simulink model "full_Model"  (R2022b)
settings: Solver=ode15s  StartTime=0.0  StopTime=400  RelTol=1e-3
InitFcn:
  | ManipulatorSetup
  | init_quad_new_leg_raibert_strategy_v2
values from neighbouring files (symbols this model uses):
  body = 'obstacle'+string(i)    [GUIWithNavigation.m]    (also in RunModel.m)
  endx = 11    [EnvironmentData.mat]    (also in Practice data.mat = 15)
  endy = 11    [EnvironmentData.mat]    (also in Practice data.mat = 14)
  floorl = 20    [EnvironmentData.mat]    (also in GUIWithNavigation.m; Practice data.mat; RunModel.m)
  floorw = 20    [EnvironmentData.mat]    (also in GUIWithNavigation.m; Practice data.mat; RunModel.m)
  planner = plannerRRTStar(ss,stateValidator)    [GUIWithNavigation.m]    (also in RunModel.m)
  startx = 3    [EnvironmentData.mat]    (also in Practice data.mat = 2)
  starty = 3    [EnvironmentData.mat]    (also in Practice data.mat = 2)
  tar1Len = 4    [EnvironmentData.mat]    (also in GUIWithNavigation.m = length(target1); Practice data.mat = 13; RunModel.m = length(target1))
  target = [3 4.43809906251 6.0940682614 6.5 6.5 7.89980588964 9.34167702197 10.6 3 4.34493388975 5.46510729784 7 ... (16 elements, 8x2)]    [EnvironmentData.mat]    (also in GUIWithNavigation.m = cat(1,target1,target2); Practice data.mat = [2 3.44057581018 5.07942513831 5.42542290116 7.21306818311 8; RunModel.m = cat(1,target1,target2))
  tarLen = 8    [EnvironmentData.mat]    (also in RunModel.m = length(target))
undefined symbols (not defined in the file or in its folder): closeFingers, ctrl, Extr_Data_LinkEndHole, grabObjectAngles, grabObjectAngles2, ground, holdFingers, homeAngles, inverseKinematicWeights, l1, l2, m1, m2, openFingers, readyAngles, X, Y, Z
libraries: sm_lib x441, nesl_utility x134, slpidlib x31, robotmaniplib x6, fl_ps_legacy_lib x6, simulink x5, fl_lib x5, Contact_Forces_Lib x4, Parts_Lib x4, sharedtransform x2, dspstat3 x1
(part 15 of 15)

== system full_Model/Manipulator2/Subsystem1/Subsystem7/Subsystem4 ==
  timeValues : Inport
  angleRange : Inport  Port=2
  currentTime : Inport  Port=3
  1-D Lookup Table : Lookup_n-D  NumberOfTableDimensions=1  BreakpointsForDimension1Source=Input port  BreakpointsForDimension1=[-5:5]  TableSource=Input port  Table=tanh([-5:5])  InternalRulePriority=Speed  RndMeth=Simplest
      settings: InputPortMap=u0,p221,p5
  anglePosition : Outport
  wires:
  timeValues/1 -> 1-D Lookup Table/3
  1-D Lookup Table/1 -> anglePosition/1
  currentTime/1 -> 1-D Lookup Table/1
  angleRange/1 -> 1-D Lookup Table/2

== system full_Model/Manipulator2/Subsystem1/Subsystem7/Subsystem5 ==
  timeValues : Inport
  angleRange : Inport  Port=2
  currentTime : Inport  Port=3
  1-D Lookup Table : Lookup_n-D  NumberOfTableDimensions=1  BreakpointsForDimension1Source=Input port  BreakpointsForDimension1=[-5:5]  TableSource=Input port  Table=tanh([-5:5])  InternalRulePriority=Speed  RndMeth=Simplest
      settings: InputPortMap=u0,p221,p5
  anglePosition : Outport
  wires:
  timeValues/1 -> 1-D Lookup Table/3
  1-D Lookup Table/1 -> anglePosition/1
  currentTime/1 -> 1-D Lookup Table/1
  angleRange/1 -> 1-D Lookup Table/2

== system full_Model/Manipulator2/Subsystem1/Subsystem7/Subsystem6 ==
  timeValues : Inport
  angleRange : Inport  Port=2
  currentTime : Inport  Port=3
  1-D Lookup Table : Lookup_n-D  NumberOfTableDimensions=1  BreakpointsForDimension1Source=Input port  BreakpointsForDimension1=[-5:5]  TableSource=Input port  Table=tanh([-5:5])  InternalRulePriority=Speed  RndMeth=Simplest
      settings: InputPortMap=u0,p221,p5
  anglePosition : Outport
  wires:
  timeValues/1 -> 1-D Lookup Table/3
  1-D Lookup Table/1 -> anglePosition/1
  currentTime/1 -> 1-D Lookup Table/1
  angleRange/1 -> 1-D Lookup Table/2

== matlab function full_Model/Controller/QuadCtrl ==
  settings: updateMethod=DISCRETE
  data: fl_ang input; tgt_ctrl_fl output; fr_ang input; rl_ang input; rr_ang input; contact_state input; body_R input; sensing_info input; tgt_ctrl_fr output; tgt_ctrl_rl output; tgt_ctrl_rr output; t input; body parameter; planner parameter; mode input; ctrl_state output; debug output; next_state input
function [tgt_ctrl_fl,tgt_ctrl_fr,tgt_ctrl_rl,tgt_ctrl_rr, ctrl_state, debug] = ...
    controller(fl_ang, fr_ang, rl_ang, rr_ang, ...
    contact_state, body_R, sensing_info, t, body, planner, mode, next_state)

%unpack sensing_info
body_vx = sensing_info(4);
body_vy = sensing_info(5);

% distance from center of mass to shoulder
fl_offset = [body.shoulder_distance;body.y_length/2+body.shoulder_size/2;0];
fr_offset = [body.shoulder_distance;-body.y_length/2-body.shoulder_size/2;0];
rl_offset = [-body.shoulder_distance;body.y_length/2+body.shoulder_size/2;0];
rr_offset = [-body.shoulder_distance;-body.y_length/2-body.shoulder_size/2;0];

%decide state and state transition helpers
persistent state;
persistent timer;
persistent timer2;
if isempty(state)
    state = 0;
end
if isempty(timer)
    timer = 0;
end
if isempty(timer2)
    timer2 = 0;
end

% init variables
           % fl fr rl rr
has_u_ctrl = [1 1 1 1];
normal_virtual_leg1 = [0;0;planner.stand_height];
normal_virtual_leg2 = [0;0;planner.stand_height];
move_fl_end_effector = normal_virtual_leg1;
move_rr_end_effector = normal_virtual_leg1;
move_fr_end_effector = normal_virtual_leg2;
move_rl_end_effector = normal_virtual_leg2;

% turning on spot mechanic
isTurning = mode == 2 || mode == 3;
%{
if isTurning
    leg_a_coef = 1; % -1/3
    leg_b_coef = 1;
else
    leg_a_coef = 1;
    leg_b_coef = 1;
end
%}
leg_a_coef = 1;
leg_b_coef = 1;

% state machine

if state == 0 % standby state
    % in this state, just do nothing, but use time to make sure that all
    % feet stands on the ground

    if contact_state(1) == 1 && contact_state(2) == 1 && contact_state(3) == 1 && contact_state(4) == 1
        %all foot on ground
        if abs(body_vx) < planner.state0_vel_thres 
            timer = timer + 1;
        else
            timer = 0;
        end
        if timer > planner.state0_trans_thres 
            state = 1;
            timer = 0;
        end
    end
elseif state == 1 % swing whole body to get a inital velocity
    timer2 = timer2 + 1;
    move_theta = planner.state0_swing_ang*sin(2*pi/planner.state0_swing_T*timer2);
    move_leg_Rx = [cos(move_theta) 0 sin(move_theta);
        0 1 0;
        -sin(move_theta) 0 cos(move_theta)];
    tgt_virtual_leg1_b = move_leg_Rx*normal_virtual_leg1;
    tgt_virtual_leg2_b = move_leg_Rx*normal_virtual_leg2;
    move_fl_end_effector = tgt_virtual_leg1_b;
    move_rr_end_effector = tgt_virtual_leg1_b;
    move_fr_end_effector = tgt_virtual_leg2_b;
    move_rl_end_effector = tgt_virtual_leg2_b;
        
    if body_vx > planner.state12_trans_speed
        timer = timer + 1;
    else
        timer = 0;
    end
    if timer > 40  %(keep a velocity larger than 0.2 for 0.1s)
        state = next_state;
        timer = 0;
        timer2 = 0;
    end

elseif state == 2 % stance virtual leg1, swing virtual leg2
    timer2 = timer2 + 1;
    if timer2 > planner.leg_swing_time %(0.5s finish movement)
        timer2 = planner.leg_swing_time;
    end
    % stance leg no u control but need to balance the body
               % fl fr rl rr
    has_u_ctrl = [0 1 1 0];
    t = timer2/planner.leg_swing_time;
%     stance_length_coeff = 0.95+0.05*(timer2/planner.leg_swing_time);
    stance_length_coeff = 0.2*t^2 - 0.2*t + 1;
    tgt_virtual_leg1_b = stance_length_coeff*normal_virtual_leg1;
    move_fl_end_effector = tgt_virtual_leg1_b;
    move_rr_end_effector = tgt_virtual_leg1_b;
    
    
    % swing leg must consider body angle 
%     move_theta = -11/180*pi*(t);
    length_coeff = 0.8*t^2-0.8*t+1;
    % move leg in x direction
    move_theta = get_move_angle(length_coeff*normal_virtual_leg2,body_vx, planner.tgt_body_vx, planner);
    
    move_leg_Rx = [cos(move_theta) 0 sin(move_theta);
        0 1 0;
        -sin(move_theta) 0 cos(move_theta)];
    move_leg_Rx2 = [cos(move_theta) 0 sin(move_theta);
        0 1 0;
        -sin(move_theta) 0 cos(move_theta)];
    tgt_virtual_leg2_a = length_coeff*move_leg_Rx2*normal_virtual_leg2;
    tgt_virtual_leg2_b = length_coeff*move_leg_Rx*normal_virtual_leg2;
    
    % move leg in y direction
    sagittal_angle = get_sagittal_angle(tgt_virtual_leg2_b,body_R, body_vy, planner);
    move_leg_Ry =[1 0 0;
                 0 cos(sagittal_angle) -sin(sagittal_angle);
                 0 sin(sagittal_angle) cos(sagittal_angle)];
    tgt_virtual_leg2_b = move_leg_Ry*tgt_virtual_leg2_b;
    tgt_virtual_leg2_a = move_leg_Ry*tgt_virtual_leg2_a;
    
    
    move_fr_end_effector = body_R'*(tgt_virtual_leg2_b+fr_offset)-fr_offset;
    if norm(move_fr_end_effector) > body.max_stretch
        move_fr_end_effector = move_fr_end_effector/norm(move_fr_end_effector)*body.max_stretch;
    end
    move_rl_end_effector = body_R'*(tgt_virtual_leg2_a+rl_offset)-rl_offset;
    if norm(move_rl_end_effector) > body.max_stretch
        move_rl_end_effector = move_rl_end_effector/norm(move_rl_end_effector)*body.max_stretch;
    end
    
    % state transition
%     if timer2 == planner.leg_swing_time
    if timer2 > 0.5*planner.leg_swing_time && contact_state(2) == 1 && contact_state(3) == 1
        timer = timer + 1;
    else
        timer = 0;
    end
    if timer > 5   % to be determined
        state = next_state;
        timer = 0;
        timer2 = 0;
    end
    
elseif state == 3 % swing virtual leg1, stance virtual leg2
    timer2 = timer2 + 1;
    if timer2 > planner.leg_swing_time %(0.5s finish movement)
        timer2 = planner.leg_swing_time;
    end
    % stance leg no u control but need to balance the body
               % fl fr rl rr
    has_u_ctrl = [1 0 0 1];
%     stance_length_coeff = 0.95+0.05*(timer2/planner.leg_swing_time);
    t = timer2/planner.leg_swing_time;
    stance_length_coeff = 0.2*t^2 - 0.2*t + 1;
    tgt_virtual_leg2_b = stance_length_coeff*normal_virtual_leg2;
    move_fr_end_effector = tgt_virtual_leg2_b;
    move_rl_end_effector = tgt_virtual_leg2_b;
    
    % swing leg must consider body angle 
    % theta is a function of forward velocity 
%     move_theta = -11/180*pi*(t);
    length_coeff = 0.8*t^2-0.8*t+1;
    move_theta = get_move_angle(length_coeff*normal_virtual_leg1,body_vx, planner.tgt_body_vx, planner);
    move_leg_Rx = [cos(move_theta*(1-2*isTurning)) 0 sin(move_theta*(1-2*isTurning));
        0 1 0;
        -sin(move_theta*(1-2*isTurning)) 0 cos(move_theta*(1-2*isTurning))];
    move_leg_Rx2 = [cos(move_theta*(1-2*isTurning)) 0 sin(move_theta*(1-2*isTurning));
        0 1 0;
        -sin(move_theta*(1-2*isTurning)) 0 cos(move_theta*(1-2*isTurning))];
    tgt_virtual_leg1_a = length_coeff*move_leg_Rx2*normal_virtual_leg1;
    tgt_virtual_leg1_b = length_coeff*move_leg_Rx*normal_virtual_leg1;
    
    % move leg in y direction
    sagittal_angle = get_sagittal_angle(tgt_virtual_leg1_b,body_R, body_vy, planner);
    move_leg_Ry =[1 0 0;
                 0 cos(sagittal_angle) -sin(sagittal_angle);
                 0 sin(sagittal_angle) cos(sagittal_angle)];
    tgt_virtual_leg1_b = move_leg_Ry*tgt_virtual_leg1_b;
    tgt_virtual_leg1_a = move_leg_Ry*tgt_virtual_leg1_a;
    
    move_fl_end_effector = body_R'*(tgt_virtual_leg1_b+fl_offset)-fl_offset;
    if norm(move_fl_end_effector) > body.max_stretch
        move_fl_end_effector = move_fl_end_effector/norm(move_fl_end_effector)*body.max_stretch;
    end
    move_rr_end_effector = body_R'*(tgt_virtual_leg1_a+rr_offset)-rr_offset;
    if norm(move_rr_end_effector) > body.max_stretch
        move_rr_end_effector = move_rr_end_effector/norm(move_rr_end_effector)*body.max_stretch;
    end
    
    % state transition
%     if timer2 == planner.leg_swing_time
    if timer2 > 0.5*planner.leg_swing_time && contact_state(1) == 1 && contact_state(4) == 1
        timer = timer + 1;
    else
        timer = 0;
    end
    if timer > 5   % to be determined
        state = next_state;
        timer = 0;
        timer2 = 0;
    end
elseif state == 4 % stabalisation
    timer2 = timer2 + 1;
    move_theta = planner.state0_swing_ang*sin(2*pi/planner.state0_swing_T*timer2);
    move_leg_Rx = [cos(move_theta) 0 sin(move_theta);
        0 1 0;
        -sin(move_theta) 0 cos(move_theta)];
    tgt_virtual_leg1_b = move_leg_Rx*normal_virtual_leg1;
    tgt_virtual_leg2_b = move_leg_Rx*normal_virtual_leg2;
    move_fl_end_effector = tgt_virtual_leg1_b;
    move_rr_end_effector = tgt_virtual_leg1_b;
    move_fr_end_effector = tgt_virtual_leg2_b;
    move_rl_end_effector = tgt_virtual_leg2_b;
        
    timer = timer + 1;
    if timer > 40  %(keep a velocity larger than 0.2 for 0.1s)
        state = next_state;
        timer = 0;
        timer2 = 0;
    end
end

%% fl to joint
[inv_s,inv_u,inv_k] = inverse_kinematics(move_fl_end_effector, body);
fl_tgt_ang_s = inv_s; 
fl_tgt_ang_u = inv_u;       
fl_tgt_ang_k = inv_k; 
tgt_ctrl_fl = [fl_tgt_ang_s;fl_tgt_ang_u;fl_tgt_ang_k;has_u_ctrl(1)];

%% fr to joint
[inv_s,inv_u,inv_k] = inverse_kinematics(move_fr_end_effector, body);
fr_tgt_ang_s = inv_s;
fr_tgt_ang_u = inv_u;
fr_tgt_ang_k = inv_k;
tgt_ctrl_fr = [fr_tgt_ang_s;fr_tgt_ang_u;fr_tgt_ang_k;has_u_ctrl(2)];

%% rl to joint
[inv_s,inv_u,inv_k] = inverse_kinematics(move_rl_end_effector, body);
rl_tgt_ang_s = inv_s;
rl_tgt_ang_u = inv_u;
rl_tgt_ang_k = inv_k;
tgt_ctrl_rl = [rl_tgt_ang_s;rl_tgt_ang_u;rl_tgt_ang_k;has_u_ctrl(3)];

%% rr to joint
[inv_s,inv_u,inv_k] = inverse_kinematics(move_rr_end_effector, body);
rr_tgt_ang_s = inv_s;
rr_tgt_ang_u = inv_u;
rr_tgt_ang_k = inv_k; 
tgt_ctrl_rr = [rr_tgt_ang_s;rr_tgt_ang_u;rr_tgt_ang_k;has_u_ctrl(4)];

ctrl_state = state;
debug = timer;

end

function move_angle = get_move_angle(virtual_leg,body_vx, tgt_body_vx, planner)

    distance = body_vx* planner.Ts/2 + planner.Kv*(tgt_body_vx-body_vx);
    
    if distance > 0.5*norm(virtual_leg)
        distance = 0.5*norm(virtual_leg);
    elseif distance < -0.5*norm(virtual_leg)
        distance = -0.5*norm(virtual_leg);
    end
    
    move_angle = asin(distance/norm(virtual_leg));
    if move_angle > 20/180*pi
        move_angle = 20/180*pi;
    elseif move_angle < -20/180*pi
        move_angle = -20/180*pi;
    end
    
end

function move_angle = get_sagittal_angle(virtual_leg,body_R, body_vy, planner)

    distance = body_vy* planner.y_Ts/2 + planner.y_Kv*(0-body_vy);  

    if distance > 0.5*norm(virtual_leg)
        distance = 0.5*norm(virtual_leg);
    elseif distance < -0.5*norm(virtual_leg)
        distance = -0.5*norm(virtual_leg);
    end
    
    move_angle = asin(distance/norm(virtual_leg));
    if move_angle > 20/180*pi
        move_angle = 20/180*pi;
    elseif move_angle < -20/180*pi
        move_angle = -20/180*pi;
    end
    
end

== stateflow chart full_Model/Controller/High Level Mode Stateflow ==
  state ResetPos
    mode=0;
    ManipTask=1;
  state Stationary
    mode=0;
    ManipTask=0;
  state Turning_Right
    mode=2;
  state Walking
    mode=1;
  state Turning_Left
    mode=3;
  Turning_Right -> ResetPos [order 2] : [resetPos==1]{pos_index=pos_index+2}
  Stationary -> ResetPos [order 2] : [resetPos==1]{pos_index=pos_index+2}
  ResetPos -> Stationary : [manipState==5]
  Walking -> ResetPos [order 4] : [resetPos==1]{pos_index=pos_index+2}
  Turning_Left -> ResetPos [order 2] : [resetPos==1]{pos_index=pos_index+2}
  (default) -> Stationary : {pos_index =2 }
  Turning_Left -> Stationary [order 1] : [delta_theta < ang_threshold]
  Turning_Right -> Stationary [order 1] : [delta_theta > -ang_threshold]
  Stationary -> Walking [order 1] : [~target_reached]
  Walking -> Stationary [order 3] : [target_reached]
      | {pos_index = pos_index + 1}
  Walking -> Turning_Right [order 2] : [delta_theta < -ang_threshold]
  Walking -> Turning_Left [order 1] : [delta_theta > ang_threshold]
  data: pos_index output =0; mode output =0; target_reached input; delta_theta input; ang_threshold local =0.2; resetPos input; ManipTask output; manipState input

== stateflow chart full_Model/Controller/Chart ==
  state PathFollowing
    resetPos=0;
  state ManipulatorTask
    resetPos=1;
  (default) -> PathFollowing
  PathFollowing -> ManipulatorTask : [pos_index==tar1Len]
  ManipulatorTask -> PathFollowing : [manipState==5]
  data: pos_index input; tar1Len input; resetPos output; manipState input

== matlab function full_Model/Manipulator2/Ball Tracking and Handling/MATLAB Function1 ==
  data: objectTransform output; x input; y input; z input; aboveObjectTransform output
function [objectTransform,aboveObjectTransform] = fcn(x,y,z)
rotTransform=[1 0 0;0 -1 0;0 0 -1];
F=rotTransform;
xline=F(1,:);
yline=F(2,:);
zline=F(3,:);
objectTransform = [ xline x;yline y;zline z+0.02;0 0 0 1];
aboveObjectTransform = [xline x;yline y;zline z+0.1;0 0 0 1];

== matlab function full_Model/Manipulator1/MATLAB Function ==
  settings: updateMethod=DISCRETE
  data: quadrupedInPosition input; errorVals input; contactForces input; state input; y output; readyAngles input; grabObjectAngles2 input; grabObjectAngles input; openFingers input; closeFingers input; holdFingers input; stateOut output; objectPosition input; aboveObjectPosition input
function [y,stateOut] = fcn(quadrupedInPosition,errorVals,contactForces,state,readyAngles,grabObjectAngles2,grabObjectAngles,openFingers,closeFingers,holdFingers,objectPosition,aboveObjectPosition)

if quadrupedInPosition == 1
    state = int16(state);

    switch state
        case 0
            y = [readyAngles;openFingers];
        case 1

            y = [aboveObjectPosition;openFingers];
        case 2
            y = [objectPosition;openFingers];
        case 3
            y = [objectPosition;closeFingers];
        case 4
            y = [aboveObjectPosition;closeFingers];
        case 5
            y = [readyAngles;closeFingers];
        otherwise
            y = zeros(13,1);
    end
    
    if state == 0 && min(errorVals) >= -0.01 && max(errorVals) <=0.01
        
        stateOut = 1;
        tic;
    elseif state == 1 && min(errorVals) >= -0.01 && max(errorVals) <=0.01 && toc >= 4
        stateOut = 2;
        tic;
    elseif state == 2 && min(errorVals) >= -0.01 && max(errorVals) <=0.01 && toc >= 0.5
        stateOut = 3;
        tic;
    elseif state == 3 && min(contactForces) >= 0.5 && toc >= 1
        toc;
        stateOut = 4;
        tic;
    elseif state == 4 && min(errorVals) >= -0.01 && max(errorVals) <=0.01 && toc >= 10
        stateOut = 5;
    elseif state == 5 && min(errorVals) >= -0.01 && max(errorVals) <=0.01
        stateOut = 5;
    else
        stateOut = double(state);
    end
else
    y = [readyAngles;openFingers];
    stateOut = 0;
end

== matlab function full_Model/Manipulator1/MATLAB Function1 ==
  data: R input; objectTransform output; x input; y input; z input; aboveObjectTransform output
function [objectTransform,aboveObjectTransform] = fcn(R,x,y,z)

objectTransform = [1 0 0 x;0 -1 0 y;0 0 -1 z+0.02;0 0 0 1];
aboveObjectTransform = [1 0 0 x;0 -1 0 y;0 0 -1 z+0.1;0 0 0 1];

== matlab function full_Model/Manipulator2/End Tracking and handling/MATLAB Function1 ==
  data: objectTransform output; x input; y input; z input; aboveObjectTransform output
function [objectTransform,aboveObjectTransform] = fcn(x,y,z)
rotTransform=[1 0 0;0 -1 0;0 0 -1];
F=rotTransform;
xline=F(1,:);
yline=F(2,:);
zline=F(3,:);
objectTransform = [ xline x;yline y;zline z+0.02;0 0 0 1];
aboveObjectTransform = [xline x;yline y;zline z+0.1;0 0 0 1];

== matlab function full_Model/Manipulator2/MATLAB Function ==
  settings: updateMethod=DISCRETE
  data: quadrupedInPosition input; errorVals input; state input; readyAngles input; openFingers input; closeFingers input; objectPosition input; aboveObjectPosition input; endPos input; aboveEndPos input; time input; y output; stateOut output; getBallPos output; getEndPos output; ballGot output
function [y,stateOut,getBallPos,getEndPos,ballGot] = fcn(quadrupedInPosition,errorVals,state,readyAngles,openFingers,closeFingers,objectPosition,aboveObjectPosition,endPos,aboveEndPos,time)

persistent startTime
if isempty(startTime)
    startTime=0;
end

threshold=0.05;
if quadrupedInPosition == 1
    state = int16(state);

    switch state
        case 0
            y = [readyAngles;openFingers];
            getBallPos=0;
            getEndPos=0;
            ballGot=0;
        case 1
            getBallPos=0;
            getEndPos=0;
            y = [aboveObjectPosition;openFingers];
            ballGot=0;
        case 2
            getBallPos=0;
            getEndPos=0;
            y = [objectPosition;openFingers];
            ballGot=0;
        case 3
            getBallPos=0;
            getEndPos=0;
            y = [objectPosition;closeFingers];
            ballGot=0;
        case 4
            getBallPos=0;
            getEndPos=0;
            y = [aboveObjectPosition;closeFingers];
            ballGot=1;
        case 5
            getBallPos=0;
            getEndPos=0;
            y = [readyAngles;closeFingers];
            ballGot=1;
        otherwise
            y = zeros(13,1);
            getBallPos=0;
            getEndPos=0;
            ballGot=0;
    end
    
    if state == 0 && min(errorVals) >= -threshold && max(errorVals) <=threshold
        getBallPos=1;
        stateOut = 1;
        startTime=time;
    elseif state == 1 && min(errorVals) >= -threshold && max(errorVals) <=threshold && (time-startTime) >= 4
        getBallPos=1;
        stateOut = 2;
        startTime=time;
    elseif state == 2  && (time-startTime) >= 4
        stateOut = 3;
        startTime=time;
    elseif state==3 && min(errorVals) >= -threshold && max(errorVals) <=threshold && (time-startTime) >= 4
        stateOut = 4;
        startTime=time;
    elseif state == 4 && min(errorVals) >= -threshold && max(errorVals) <=threshold && (time-startTime) >= 4
        stateOut = 5;
        startTime=time;
    elseif state == 5 && min(errorVals) >= -threshold && max(errorVals) <=threshold && (time-startTime)>=4
        stateOut = 5;
    else
        stateOut = double(state);
    end

elseif quadrupedInPosition == 2

    switch state
        case 5
            y = [readyAngles;closeFingers];
            getBallPos=0;
            getEndPos=0;
            ballGot=1;
        case 6
            getBallPos=0;
            getEndPos=0;
            y = [aboveEndPos;closeFingers];
            ballGot=1;
        case 7
            getBallPos=0;
            getEndPos=0;
            y = [endPos;closeFingers];
            ballGot=1;
        case 8
            getBallPos=0;
            getEndPos=0;
            y = [endPos;openFingers];
            ballGot=1;
        case 9
            getBallPos=0;
            getEndPos=0;
            y = [aboveEndPos;openFingers];
            ballGot=0;
        case 10
            getBallPos=0;
            getEndPos=0;
            y = [readyAngles;openFingers];
            ballGot=0;
        case 11
            getBallPos=0;
            getEndPos=0;
            y = [readyAngles;openFingers];
            ballGot=0;
        otherwise
            y = zeros(13,1);
            getBallPos=0;
            getEndPos=0;
            ballGot=0;
    end
    if state == 5 && min(errorVals) >= -threshold && max(errorVals) <=threshold
        stateOut = 6;
        startTime=time;
    elseif state == 6 && min(errorVals) >= -threshold && max(errorVals) <=threshold && (time-startTime) >= 4
        getEndPos=1;
        stateOut = 7;
        startTime=time;
    elseif state == 7  && (time-startTime) >= 4
        stateOut = 8;
        startTime=time;
    elseif state==8 && min(errorVals) >= -threshold && max(errorVals) <=threshold && (time-startTime) >= 5
        stateOut = 9;
        startTime=time;
    elseif state == 9 && min(errorVals) >= -threshold && max(errorVals) <=threshold && (time-startTime) >= 10
        stateOut = 10;
        startTime=time;
    elseif state == 10 && min(errorVals) >= -threshold && max(errorVals) <=threshold && (time-startTime)>=4
        stateOut = 11;
        startTime=time;
    elseif state == 11 && min(errorVals) >= -threshold && max(errorVals) <=threshold && (time-startTime)>=4
        stateOut = 11;
    else
        stateOut = double(state);
    end
else
    y = [readyAngles;openFingers];
    stateOut = 0;
    getBallPos=0;
    getEndPos=0;
    ballGot=0;
end

== matlab function full_Model/Manipulator2/Subsystem1/Manipulator interpolator ==
  settings: updateMethod=DISCRETE
  data: desiredAngles input size=[7  1]; angleRangeOut output size=[1 14]; currentAngles input size=[7 1]; timeRangeOut output size=[1 14]; time input; debug output
function [angleRangeOut,timeRangeOut,debug]  = manipInterp(desiredAngles,currentAngles,time)

persistent beginState
persistent ready1
persistent ready2
persistent ready3
persistent ready4
persistent ready5
persistent ready6
persistent ready7

% persistent interval
persistent startTime
persistent angleRange
persistent timeRange

if isempty(beginState)
    beginState=transpose(currentAngles);
end

% if isempty(interval)
%     interval=0.01;
% end
if isempty(startTime)
    startTime=10;
end
if isempty(angleRange)
    angleRange=[transpose(currentAngles),transpose(currentAngles)];
end
if isempty(timeRange)
    timeRange=[ones(1,7)*0,ones(1,7)*600];
end
if isempty(ready1)
    ready1=0;
end
if isempty(ready2)
    ready2=0;
end
if isempty(ready3)
    ready3=0;
end
if isempty(ready4)
    ready4=0;
end
if isempty(ready5)
    ready5=0;
end
if isempty(ready6)
    ready6=0;
end
if isempty(ready7)
    ready7=0;
end

%timeSteps=0.01;
transferTime=3;
%calcTime=timeSteps/transferTime;
angleDif=transpose(abs(desiredAngles-currentAngles));
threshold=0.01;
TcurrentAngles=transpose(currentAngles);
if angleDif(1)>=threshold||angleDif(2)>=threshold||angleDif(3)>=threshold||angleDif(4)>=threshold||angleDif(5)>=threshold||angleDif(6)>=threshold||angleDif(7)>=threshold
    if ready1==0&&ready2==0&&ready3==0&&ready4==0&&ready5==0&&ready6==0&&ready7==0
        beginState=transpose(currentAngles);
        %interval=((desiredAngles-beginState)./calcTime);
        startTime=time;
        ready1=1;
        ready2=1;
        ready3=1;
        ready4=1;
        ready5=1;
        ready6=1;
        ready7=1;
        endTime=transferTime+startTime;
        timeRange=[ones(1,7)*startTime,ones(1,7)*endTime];
        angleRange=[beginState,transpose(desiredAngles)];
    end       
end

if angleDif(1)<=threshold
    ready1=0;
    timeRange(1)=0;
    timeRange(8)=600;
    angleRange(1)=TcurrentAngles(1);
    angleRange(8)=TcurrentAngles(1);
end
if angleDif(2)<=threshold
    ready2=0;
    timeRange(2)=0;
    timeRange(9)=600;
    angleRange(2)=TcurrentAngles(2);
    angleRange(9)=TcurrentAngles(2);
end
if angleDif(3)<=threshold
    ready3=0;
    timeRange(3)=0;
    timeRange(10)=600;
    angleRange(3)=TcurrentAngles(3);
    angleRange(10)=TcurrentAngles(3);
end
if angleDif(4)<=threshold
    ready4=0;
    timeRange(4)=0;
    timeRange(11)=600;
    angleRange(4)=TcurrentAngles(4);
    angleRange(11)=TcurrentAngles(4);
end
if angleDif(5)<=threshold
    ready5=0;
    timeRange(5)=0;
    timeRange(12)=600;
    angleRange(5)=TcurrentAngles(5);
    angleRange(12)=TcurrentAngles(5);
end
if angleDif(6)<=threshold
    ready6=0;
    timeRange(6)=0;
    timeRange(13)=600;
    angleRange(6)=TcurrentAngles(6);
    angleRange(13)=TcurrentAngles(6);
end
if angleDif(7)<=threshold
    ready7=0;
    timeRange(7)=0;
    timeRange(14)=600;
    angleRange(7)=TcurrentAngles(7);
    angleRange(14)=TcurrentAngles(7);
end

angleRangeOut=angleRange;
timeRangeOut=timeRange;
debug=angleDif;

== matlab function full_Model/Controller/MATLAB Function1 ==
  settings: updateMethod=DISCRETE
  data: go input; mode output; targets input; tar1Len input; tarLen input; x input; y input; angle input; done output
function [mode,done] = broadside(go,targets,tar1Len,tarLen,x,y,angle)

persistent targetAssigned
if isempty(targetAssigned)
    targetAssigned=0;
end

persistent broadTarget
if isempty(broadTarget)
    broadTarget=[0,0];
end

persistent points
if isempty(points)
    points=0;
end

persistent point1
if isempty(point1)
    point1=[0,0];
end

persistent point2
if isempty(point2)
    point2=[0,0];
end

persistent currentTarget
if isempty(currentTarget)
    currentTarget=[0,0];
end


if go==1||go==2
    if targetAssigned==0
        if go==1
            broadTarget=targets(tar1Len,:);
        elseif go==2
            broadTarget=targets(tarLen,:);
        end
        if y>broadTarget(2)
            spacing=1;
        else
            spacing=-1;
        end
        if x>broadTarget(1)
            points=2;
            point1=[x,broadTarget(2)+spacing];
            point2=[broadTarget(1),broadTarget(2)+spacing];
        else
            points=1;
            point1=[broadTarget(1),broadTarget(2)+spacing];
        end
        currentTarget=point1;
        targetAssigned=1;
    end
    delta=currentTarget-[x,y];
    deltaDist=sqrt(delta(1).^2+delta(2).^2);
    targetAngle=atan2(delta(2),delta(1));
    deltaAngle=targetAngle-angle;
    if abs(deltaDist)>=0.1
        if deltaAngle<-0.1
            %disp('im left')
            %turn right
            mode=2;

        elseif deltaAngle>0.1
            %disp('im right')
            %turn left
            mode=3;
        else
            disp('im forward')
            mode=1;
        end
        done=0;
    else
        if (currentTarget-point1)*[1;1]==0&&points==1
            currentTarget=[broadTarget(1),broadTarget(2)];
            done=0;
        elseif (currentTarget-point1)*[1;1]==0&&points==2
            currentTarget=point2;
            done=0;
        elseif (currentTarget-point2)*[1;1]==0
            currentTarget=[broadTarget(1),broadTarget(2)];
            done=0;
        else
            done=1;
        end
        mode=0;
    end
else
    targetAssigned=0;
    done=0;
    mode=0;
end

== stateflow chart full_Model/Controller/Subsystem/Chart ==
  state PathFollowing
    endSim=false;
    resetPos=0;
  state ManipulatorTask1
    resetPos=1;
  state PathFollowing2
    resetPos=0;
  state ManipulatorTask2
    resetPos=2;
  state EndSim
    resetPos=0;
    endSim=true;
  (default) -> PathFollowing
  PathFollowing -> ManipulatorTask1 : [abs(target(tar1Len,1))-x<=1 || abs(target(tar1Len,2)-y<=1)]{posToSkip=tar1Len-pos_index}
  ManipulatorTask1 -> PathFollowing2 : [manipState>=5]
  PathFollowing2 -> ManipulatorTask2 : [abs(target(tarLen,1))-x<=1 || abs(target(tarLen,2)-y<=1)]
  ManipulatorTask2 -> EndSim : [manipState>=11]
  data: tar1Len input; resetPos output; manipState input; tarLen input; targetReached input; endSim output; check input; target input; y input; posToSkip output; x input; pos_index input

== stateflow chart full_Model/Controller/High Level Mode Stateflow2 ==
  state ManipTask1
    ManipTask=1;
  state Broadside
    broadside=1;
  note: 0.35
  note: 1
  state ResetPos1
    mode=0;
  state Stationary
    mode=0;
  state Turning_Left
    mode=3;
  state Turning_Right
    mode=2;
  state Walking
    mode=1;
  state ResetPos2
    mode=0;
  state Broadside1
    broadside=2;
  state ManipTask2
    ManipTask=2;
  ManipTask1 -> Stationary : [resetPos==0]
  Broadside -> ManipTask1 : [broadFinished==1&&stopped]{broadside=0}
  ResetPos1 -> Broadside : [stopped]{pos_index=pos_index+1+posToSkip}
  Turning_Right -> ResetPos1 [order 2] : [resetPos==1]
  Stationary -> ResetPos1 [order 2] : [resetPos==1]
  Walking -> ResetPos1 [order 5] : [resetPos==1]
  Turning_Left -> ResetPos1 [order 3] : [resetPos==1]
  Stationary -> Stationary [order 3] : [target_reached&&pos_index~=tarLen]
      | {pos_index = pos_index + 1}
  (default) -> Stationary : {pos_index =2;bodyMode=0}
  Turning_Left -> Stationary [order 1] : [delta_theta < ang_threshold]
  Turning_Right -> Stationary [order 1] : [delta_theta > -ang_threshold]
  Walking -> Stationary [order 3] : [target_reached&&pos_index~=tarLen]
      | {pos_index = pos_index + 1}
  Stationary -> ResetPos2 [order 4] : [resetPos==2]
  Stationary -> Walking [order 1] : [~target_reached]
  Walking -> Turning_Left [order 1] : [delta_theta > ang_threshold]
  Walking -> Turning_Right [order 2] : [delta_theta < -ang_threshold]
  Turning_Left -> ResetPos2 [order 2] : [resetPos==2]
  Turning_Right -> ResetPos2 [order 3] : [resetPos==2]
  Walking -> ResetPos2 [order 4] : [resetPos==2]
  ResetPos2 -> Broadside1 : [stopped]
  Broadside1 -> ManipTask2 : [broadFinished==1&&stopped]{broadside=0}
  data: pos_index output =0; mode output =0; target_reached input; delta_theta input; ang_threshold local =0.2; resetPos input; ManipTask output; stopped input; bodyMode output; tarLen input; broadside output; broadFinished input; posToSkip input

== stateflow chart full_Model/Controller/State Transitions ==
  state Initilisation
    next_state = 1;
  state Walking_Phase_fr_rl
    next_state = 2;
  state Stationary
    next_state = 4;
  state Walking_Phase_fl_rr
    next_state = 3;
  (default) -> Initilisation
  Initilisation -> Stationary : [ctrl_state==next_state]
  Stationary -> Walking_Phase_fr_rl : [mode >= 1 && ctrl_state == next_state]
  Walking_Phase_fl_rr -> Walking_Phase_fr_rl [order 2] : [ctrl_state == next_state]
  Walking_Phase_fr_rl -> (junction 49) [order 1] : [mode == 0]
  Walking_Phase_fr_rl -> Walking_Phase_fl_rr [order 2] : [ctrl_state == next_state]
  (junction 49) -> Stationary
  Walking_Phase_fl_rr -> (junction 49) [order 1] : [mode == 0]
  data: ctrl_state input =0; mode input =0; next_state output
